simulink model "fused_model"  (R2014b)
settings: Solver=FixedStepAuto  StartTime=0.0  StopTime=100  FixedStep=0.01  RelTol=1e-3
values from neighbouring files (symbols this model uses):
  alpha_AoA = [0 1 2 3 4 5 6 7 8 9 10 11 ... (273 elements, 91x3)]    [alpha_Cd_Cl.mat]    (also in simdata_fused.mat)
  RPM_vs_Throttle = [0 2 4 6 8 10 12 14 16 18 20 22 ... (102 elements, 51x2)]    [RPM_Throttle.mat]    (also in simdata_fused.mat)
  Thrust_vs_PWM = [1100 1110 1120 1130 1140 1150 1160 1170 1180 1190 1200 1210 ... (243 elements, 81x3)]    [Thrust_PWM.mat]    (also in simdata_fused.mat)
  Thrust_vs_RPM = [0 184.4694179 362.7257873 540.6451661 718.059059 894.7989709 1070.696406 1245.58287 1419.289867 1591.648901 1762.491478 1931.649102 ... (102 elements, 51x2)]    [Thrust_RPM.mat]    (also in simdata_fused.mat)
  Torque_vs_RPM = [0 184.4694179 362.7257873 540.6451661 718.059059 894.7989709 1070.696406 1245.58287 1419.289867 1591.648901 1762.491478 1931.649102 ... (102 elements, 51x2)]    [Torque_RPM.mat]    (also in simdata_fused.mat)
libraries: simulink x2
settings Model: Creator=abhij  LastModifiedBy=harsha_home
settings DataIOCC: LimitDataPoints=off  SaveFormat=Dataset
settings OptimizationCC: UseDivisionForNetSlopeComputation=off  SimCompilerOptimization=off
settings DebuggingCC: SolverPrmCheckMsg=none  FrameProcessingCompatibilityMsg=error
settings HardwareCC: ProdBitPerPointer=64  ProdLargestAtomicFloat=Float  ProdIntDivRoundTo=Zero  ProdEndianess=LittleEndian  ProdWordSize=64  ProdHWDeviceType=Intel->x86-64 (Windows64)
settings ModelReferenceCC: PropagateSignalLabelsOutOfModel=on
settings RTWCC: RTWCompilerOptimization=off
settings ConfigComp: CovMetricSettings=dw  CovHtmlReporting=on  CovSaveCumulativeToWorkspaceVar=on  CovSaveSingleToWorkspaceVar=on  CovExternalEMLEnable=off

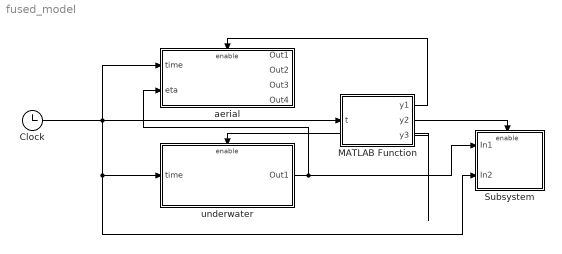
== system fused_model ==
  Clock : Clock
  MATLAB Function : MATLAB Function  TreatAsAtomicUnit=on
  Subsystem : Subsystem
  aerial : Subsystem
  underwater : Subsystem
  wires:
  Clock/1 -> aerial/1(time), Subsystem/2(In2), underwater/1(time), MATLAB Function/1(t)
  MATLAB Function/1(y1) -> aerial/Enable
  underwater/1(Out1) -> Subsystem/1(In1), aerial/2(eta)
  MATLAB Function/3(y3) -> underwater/Enable
  MATLAB Function/2(y2) -> Subsystem/Enable

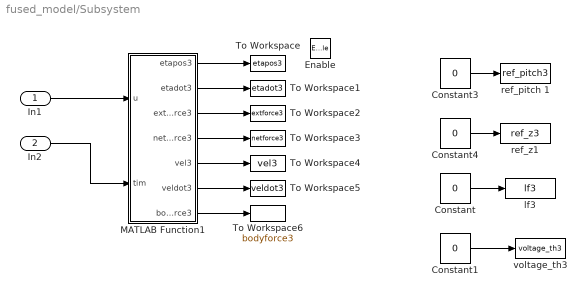
== system fused_model/Subsystem ==
  In1 : Inport
  In2 : Inport  Port=2
  Enable : EnablePort
  Constant{,1,3..4} (4 alike) : Constant  Value=0
  MATLAB Function1 : MATLAB Function  TreatAsAtomicUnit=on
  To Workspace : ToWorkspace  VariableName=etapos3  SaveFormat=Timeseries  SampleTime=-1
  To Workspace1 : ToWorkspace  VariableName=etadot3  SaveFormat=Timeseries  SampleTime=-1
  To Workspace2 : ToWorkspace  VariableName=extforce3  SaveFormat=Timeseries  SampleTime=-1
  To Workspace3 : ToWorkspace  VariableName=netforce3  SaveFormat=Timeseries  SampleTime=-1
  To Workspace4 : ToWorkspace  VariableName=vel3  SaveFormat=Timeseries  SampleTime=-1
  To Workspace5 : ToWorkspace  VariableName=veldot3  SaveFormat=Timeseries  SampleTime=-1
  To Workspace6 : ToWorkspace  VariableName=bodyforce3  SaveFormat=Timeseries  SampleTime=-1
  "lf3 " : ToWorkspace  VariableName=lf3  SaveFormat=Timeseries  SampleTime=-1
  ref_pitch 1 : ToWorkspace  VariableName=ref_pitch3  SaveFormat=Timeseries  SampleTime=-1
  ref_z1 : ToWorkspace  VariableName=ref_z3  SaveFormat=Timeseries  SampleTime=-1
  "voltage_th3 " : ToWorkspace  VariableName=voltage_th3  SaveFormat=Timeseries  SampleTime=-1
  wires:
  In1/1 -> MATLAB Function1/1(u)
  In2/1 -> MATLAB Function1/2(tim)
  MATLAB Function1/1(etapos3) -> To Workspace/1
  MATLAB Function1/2(etadot3) -> To Workspace1/1
  MATLAB Function1/3(extforce3) -> To Workspace2/1
  MATLAB Function1/4(netforce3) -> To Workspace3/1
  MATLAB Function1/5(vel3) -> To Workspace4/1
  MATLAB Function1/6(veldot3) -> To Workspace5/1
  MATLAB Function1/7(bodyforce3) -> To Workspace6/1
  Constant/1 -> "lf3 "/1
  Constant1/1 -> "voltage_th3 "/1
  Constant3/1 -> ref_pitch 1/1
  Constant4/1 -> ref_z1/1

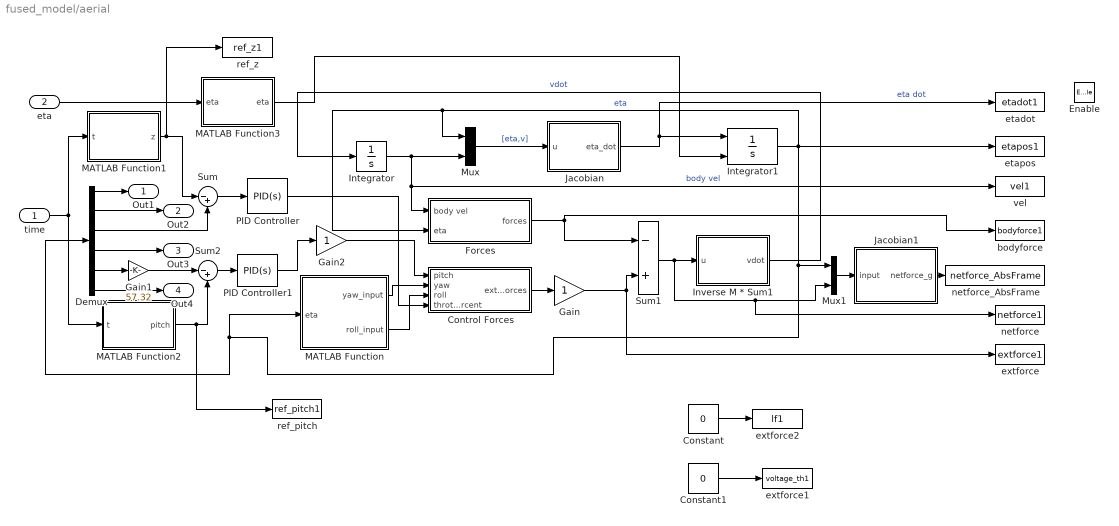
== system fused_model/aerial ==
  time : Inport
  eta : Inport  Port=2
  Enable : EnablePort
  Constant : Constant  Value=0
  Constant1 : Constant  Value=0
  Control Forces : Subsystem
  Demux : Demux  Outputs=6
  Forces : Subsystem
  Gain : Gain
  Gain1 : Gain  Gain=57.32
  Gain2 : Gain
  Integrator : Integrator  InitialCondition=[0;0;0;0;0;0]
  Integrator1 : Integrator  InitialConditionSource=external  InitialCondition=[0;0;0;0;0;0]
  Inverse M * Sum1 : MATLAB Function  TreatAsAtomicUnit=on
  Jacobian : MATLAB Function  TreatAsAtomicUnit=on
  Jacobian1 : MATLAB Function  TreatAsAtomicUnit=on
  MATLAB Function : MATLAB Function  TreatAsAtomicUnit=on
  MATLAB Function1 : MATLAB Function  TreatAsAtomicUnit=on
  MATLAB Function2 : MATLAB Function  TreatAsAtomicUnit=on
  MATLAB Function3 : MATLAB Function  TreatAsAtomicUnit=on
  Mux : Mux  Inputs=2
  Mux1 : Mux  Inputs=2
  PID Controller : simulink/Continuous/PID Controller  Controller=PID  TimeDomain=Continuous-time  SampleTime=-1  IntegratorMethod=Forward Euler  FilterMethod=Forward Euler  Form=Parallel  P=1  I=1  D=0  N=100  InitialConditionSource=internal  InitialConditionForIntegrator=0  InitialConditionForFilter=0  ExternalReset=none  LimitOutput=off  UpperSaturationLimit=inf  LowerSaturationLimit=-inf  LinearizeAsGain=on  AntiWindupMode=none  Kb=1  TrackingMode=off  Kt=1  PParamMin=[]  PParamMax=[]  IParamMin=[]  IParamMax=[]  DParamMin=[]  DParamMax=[]  NParamMin=[]  NParamMax=[]  KbParamMin=[]  KbParamMax=[]  KtParamMin=[]  KtParamMax=[]  POutMin=[]  POutMax=[]  IOutMin=[]  IOutMax=[]  DOutMin=[]  DOutMax=[]  NOutMin=[]  NOutMax=[]  KbOutMin=[]  KbOutMax=[]  KtOutMin=[]  KtOutMax=[]  IntegratorOutMin=[]  IntegratorOutMax=[]  FilterOutMin=[]  FilterOutMax=[]  SumOutMin=[]  SumOutMax=[]  SumI1OutMin=[]  SumI1OutMax=[]  SumI2OutMin=[]  SumI2OutMax=[]  SumI3OutMin=[]  SumI3OutMax=[]  SumDOutMin=[]  SumDOutMax=[]  SaturationOutMin=[]  SaturationOutMax=[]  IntegratorContinuousStateAttributes=''  IntegratorStateMustResolveToSignalObject=off  IntegratorRTWStateStorageClass=Auto  FilterContinuousStateAttributes=''  FilterStateMustResolveToSignalObject=off  FilterRTWStateStorageClass=Auto  DifferentiatorICPrevScaledInput=0  DifferentiatorOutMin=[]  DifferentiatorOutMax=[]  UseFilter=on
  PID Controller1 : simulink/Continuous/PID Controller  Controller=PID  TimeDomain=Continuous-time  SampleTime=-1  IntegratorMethod=Forward Euler  FilterMethod=Forward Euler  Form=Parallel  P=1  I=1  D=0  N=100  InitialConditionSource=internal  InitialConditionForIntegrator=0  InitialConditionForFilter=0  ExternalReset=none  LimitOutput=off  UpperSaturationLimit=inf  LowerSaturationLimit=-inf  LinearizeAsGain=on  AntiWindupMode=none  Kb=1  TrackingMode=off  Kt=1  PParamMin=[]  PParamMax=[]  IParamMin=[]  IParamMax=[]  DParamMin=[]  DParamMax=[]  NParamMin=[]  NParamMax=[]  KbParamMin=[]  KbParamMax=[]  KtParamMin=[]  KtParamMax=[]  POutMin=[]  POutMax=[]  IOutMin=[]  IOutMax=[]  DOutMin=[]  DOutMax=[]  NOutMin=[]  NOutMax=[]  KbOutMin=[]  KbOutMax=[]  KtOutMin=[]  KtOutMax=[]  IntegratorOutMin=[]  IntegratorOutMax=[]  FilterOutMin=[]  FilterOutMax=[]  SumOutMin=[]  SumOutMax=[]  SumI1OutMin=[]  SumI1OutMax=[]  SumI2OutMin=[]  SumI2OutMax=[]  SumI3OutMin=[]  SumI3OutMax=[]  SumDOutMin=[]  SumDOutMax=[]  SaturationOutMin=[]  SaturationOutMax=[]  IntegratorContinuousStateAttributes=''  IntegratorStateMustResolveToSignalObject=off  IntegratorRTWStateStorageClass=Auto  FilterContinuousStateAttributes=''  FilterStateMustResolveToSignalObject=off  FilterRTWStateStorageClass=Auto  DifferentiatorICPrevScaledInput=0  DifferentiatorOutMin=[]  DifferentiatorOutMax=[]  UseFilter=on
  Sum : Sum  Inputs=|-+
  Sum1 : Sum  Inputs=-+
  Sum2 : Sum  Inputs=|-+
  bodyforce : ToWorkspace  VariableName=bodyforce1  SaveFormat=Timeseries  SampleTime=-1
  etadot : ToWorkspace  VariableName=etadot1  SaveFormat=Timeseries  SampleTime=-1
  etapos : ToWorkspace  VariableName=etapos1  SaveFormat=Timeseries  SampleTime=-1
  extforce : ToWorkspace  VariableName=extforce1  SaveFormat=Timeseries  SampleTime=-1
  extforce1 : ToWorkspace  VariableName=voltage_th1  SaveFormat=Timeseries  SampleTime=-1
  extforce2 : ToWorkspace  VariableName=lf1  SaveFormat=Timeseries  SampleTime=-1
  netforce : ToWorkspace  VariableName=netforce1  SaveFormat=Timeseries  SampleTime=-1
  netforce_AbsFrame : ToWorkspace  VariableName=netforce_AbsFrame  SaveFormat=Timeseries  SampleTime=-1
  "ref_pitch " : ToWorkspace  VariableName=ref_pitch1  SaveFormat=Timeseries  SampleTime=-1
  ref_z : ToWorkspace  VariableName=ref_z1  SaveFormat=Timeseries  SampleTime=-1
  vel : ToWorkspace  VariableName=vel1  SaveFormat=Timeseries  SampleTime=-1
  Out1 : Outport
  Out2 : Outport  Port=2
  Out3 : Outport  Port=3
  Out4 : Outport  Port=4
  wires:
  MATLAB Function/1(yaw_input) -> Control Forces/2(yaw)
  time/1 -> MATLAB Function2/1(t), MATLAB Function1/1(t)
  Jacobian/1(eta_dot) -> etadot/1, Integrator1/1  "eta dot"
  Gain2/1 -> Control Forces/1(pitch)
  MATLAB Function/2(roll_input) -> Control Forces/3(roll)
  PID Controller1/1 -> Gain2/1
  Demux/3 -> Sum/2
  Sum1/1 -> netforce/1, Mux1/2, Inverse M * Sum1/1(u)
  MATLAB Function2/1(pitch) -> "ref_pitch "/1, Sum2/2
  PID Controller/1 -> Control Forces/4(throttle percent)
  Jacobian1/1(netforce_g) -> netforce_AbsFrame/1
  Sum2/1 -> PID Controller1/1
  Mux/1 -> Jacobian/1(u)  "[eta,v]"
  Gain/1 -> extforce/1, Sum1/2
  MATLAB Function1/1(z) -> ref_z/1, Sum/1
  Control Forces/1(external forces) -> Gain/1
  Sum/1 -> PID Controller/1
  Integrator/1 -> vel/1, Forces/1(body vel), Mux/2  "body vel"
  Integrator1/1 -> Forces/2(eta), Mux/1, Demux/1, MATLAB Function/1(eta), Mux1/1, etapos/1  "eta"
  Forces/1(forces) -> Sum1/1, bodyforce/1
  Mux1/1 -> Jacobian1/1(input)
  Demux/5 -> Gain1/1
  Gain1/1 -> Sum2/1
  eta/1 -> MATLAB Function3/1("eta ")
  Inverse M * Sum1/1(vdot) -> Integrator/1  "vdot"
  Demux/1 -> Out1/1
  Demux/2 -> Out2/1
  Demux/4 -> Out3/1
  Demux/6 -> Out4/1
  MATLAB Function3/1(eta) -> Integrator1/2
  Constant/1 -> extforce2/1
  Constant1/1 -> extforce1/1

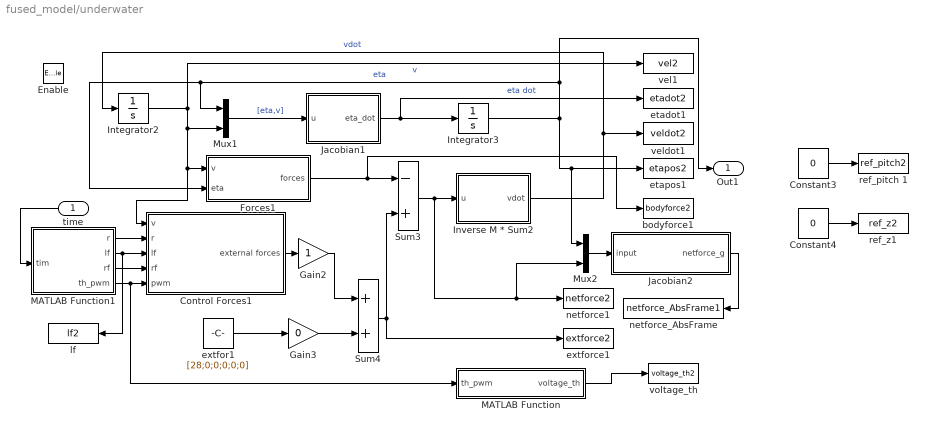
== system fused_model/underwater ==
  time : Inport
  Enable : EnablePort
  Constant3 : Constant  Value=0
  Constant4 : Constant  Value=0
  Control Forces1 : Subsystem
  Forces1 : Subsystem
  Gain2 : Gain
  Gain3 : Gain  Gain=0
  Integrator2 : Integrator  InitialCondition=[0;0;0;0;0;0]
  Integrator3 : Integrator  InitialCondition=[0;0;5;0;0;0]
  Inverse M * Sum2 : MATLAB Function  TreatAsAtomicUnit=on
  Jacobian1 : MATLAB Function  TreatAsAtomicUnit=on
  Jacobian2 : MATLAB Function  TreatAsAtomicUnit=on
  MATLAB Function : MATLAB Function  TreatAsAtomicUnit=on
  MATLAB Function1 : MATLAB Function  TreatAsAtomicUnit=on
  Mux1 : Mux  Inputs=2
  Mux2 : Mux  Inputs=2
  Sum3 : Sum  Inputs=-+
  Sum4 : Sum
  bodyforce1 : ToWorkspace  VariableName=bodyforce2  SaveFormat=Timeseries  SampleTime=-1
  etadot1 : ToWorkspace  VariableName=etadot2  SaveFormat=Timeseries  SampleTime=-1
  etapos1 : ToWorkspace  VariableName=etapos2  SaveFormat=Timeseries  SampleTime=-1
  extfor1 : Constant  Value=[28;0;0;0;0;0]
  extforce1 : ToWorkspace  VariableName=extforce2  SaveFormat=Timeseries  SampleTime=-1
  lf : ToWorkspace  VariableName=lf2  SaveFormat=Timeseries  SampleTime=-1
  netforce1 : ToWorkspace  VariableName=netforce2  SaveFormat=Timeseries  SampleTime=-1
  netforce_AbsFrame : ToWorkspace  VariableName=netforce_AbsFrame1  SaveFormat=Timeseries  SampleTime=-1
  ref_pitch 1 : ToWorkspace  VariableName=ref_pitch2  SaveFormat=Timeseries  SampleTime=-1
  ref_z1 : ToWorkspace  VariableName=ref_z2  SaveFormat=Timeseries  SampleTime=-1
  vel1 : ToWorkspace  VariableName=vel2  SaveFormat=Timeseries  SampleTime=-1
  veldot1 : ToWorkspace  VariableName=veldot2  SaveFormat=Timeseries  SampleTime=-1
  "voltage_th " : ToWorkspace  VariableName=voltage_th2  SaveFormat=Timeseries  SampleTime=-1
  Out1 : Outport
  wires:
  Integrator2/1 -> vel1/1, Forces1/1(v), Control Forces1/1(v), Mux1/2  "v"
  Mux1/1 -> Jacobian1/1(u)  "[eta,v]"
  Jacobian1/1(eta_dot) -> etadot1/1, Integrator3/1  "eta dot"
  Integrator3/1 -> Mux2/1, etapos1/1, Out1/1, Forces1/2(eta), Mux1/1  "eta"
  Sum3/1 -> netforce1/1, Mux2/2, Inverse M * Sum2/1(u)
  Forces1/1(forces) -> Sum3/1, bodyforce1/1
  Control Forces1/1(external forces) -> Gain2/1
  Gain2/1 -> Sum4/1
  Gain3/1 -> Sum4/2
  extfor1/1 -> Gain3/1
  Sum4/1 -> Sum3/2, extforce1/1
  Mux2/1 -> Jacobian2/1(input)
  Jacobian2/1(netforce_g) -> netforce_AbsFrame/1
  Inverse M * Sum2/1(vdot) -> Integrator2/1, veldot1/1  "vdot"
  MATLAB Function1/1(r) -> Control Forces1/2(r)
  MATLAB Function1/2(lf) -> Control Forces1/3(lf), lf/1
  MATLAB Function1/3(rf) -> Control Forces1/4(rf)
  time/1 -> MATLAB Function1/1(tim)
  MATLAB Function1/4(th_pwm) -> MATLAB Function/1(th_pwm), Control Forces1/5("pwm ")
  MATLAB Function/1(voltage_th) -> "voltage_th "/1
  Constant3/1 -> ref_pitch 1/1
  Constant4/1 -> ref_z1/1

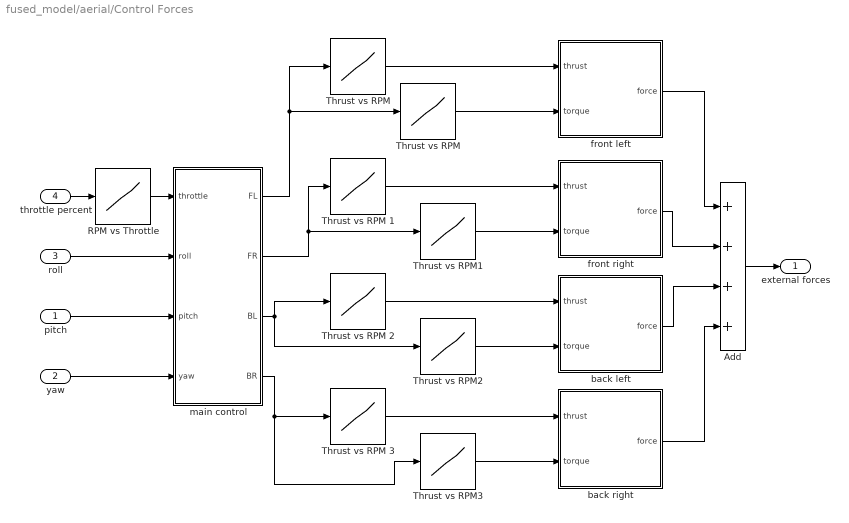
== system fused_model/aerial/Control Forces ==
  pitch : Inport
  yaw : Inport  Port=2
  roll : Inport  Port=3
  throttle percent : Inport  Port=4
  Add : Sum  Inputs=4
  "RPM vs Throttle " : Lookup_n-D  NumberOfTableDimensions=1  BreakpointsForDimension1=RPM_vs_Throttle(:,1)  Table=RPM_vs_Throttle(:,2)  InternalRulePriority=Speed  RndMeth=Simplest  InputSameDT=on
  Thrust vs RPM{,1..3} (4 alike) : Lookup_n-D  NumberOfTableDimensions=1  BreakpointsForDimension1=Torque_vs_RPM(:,1)  Table=Torque_vs_RPM(:,2)  InternalRulePriority=Speed  RndMeth=Simplest  InputSameDT=on
  Thrust vs RPM {,1..3} (4 alike) : Lookup_n-D  NumberOfTableDimensions=1  BreakpointsForDimension1=Thrust_vs_RPM(:,1)  Table=Thrust_vs_RPM(:,2)  InternalRulePriority=Speed  RndMeth=Simplest  InputSameDT=on
  back left : MATLAB Function  TreatAsAtomicUnit=on
  back right : MATLAB Function  TreatAsAtomicUnit=on
  front left : MATLAB Function  TreatAsAtomicUnit=on
  front right : MATLAB Function  TreatAsAtomicUnit=on
  main control : MATLAB Function  TreatAsAtomicUnit=on
  external forces : Outport
  wires:
  front left/1(force) -> Add/1
  front right/1(force) -> Add/2
  back left/1(force) -> Add/3
  back right/1(force) -> Add/4
  main control/1(FL) -> Thrust vs RPM/1, "Thrust vs RPM "/1
  main control/2(FR) -> Thrust vs RPM 1/1, Thrust vs RPM1/1
  main control/3(BL) -> Thrust vs RPM2/1, Thrust vs RPM 2/1
  main control/4(BR) -> Thrust vs RPM3/1, Thrust vs RPM 3/1
  throttle percent/1 -> "RPM vs Throttle "/1
  roll/1 -> main control/2(roll)
  pitch/1 -> main control/3(pitch)
  yaw/1 -> main control/4(yaw)
  "RPM vs Throttle "/1 -> main control/1(throttle)
  Thrust vs RPM/1 -> front left/2(torque)
  Thrust vs RPM1/1 -> front right/2(torque)
  Thrust vs RPM2/1 -> back left/2(torque)
  Thrust vs RPM3/1 -> back right/2(torque)
  "Thrust vs RPM "/1 -> front left/1(thrust)
  Thrust vs RPM 1/1 -> front right/1(thrust)
  Thrust vs RPM 2/1 -> back left/1(thrust)
  Thrust vs RPM 3/1 -> back right/1(thrust)
  Add/1 -> external forces/1

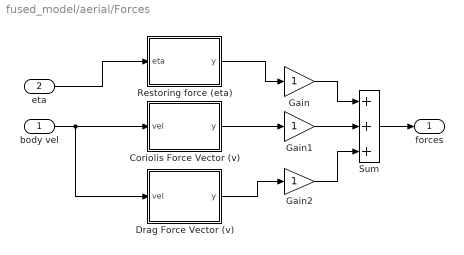
== system fused_model/aerial/Forces ==
  body vel : Inport
  eta : Inport  Port=2
  Coriolis Force Vector (v) : MATLAB Function  TreatAsAtomicUnit=on
  Drag Force Vector (v) : MATLAB Function  TreatAsAtomicUnit=on
  Gain : Gain
  Gain1 : Gain
  Gain2 : Gain
  Restoring force (eta) : MATLAB Function  TreatAsAtomicUnit=on
  Sum : Sum  Inputs=+++
  forces : Outport
  wires:
  Restoring force (eta)/1(y) -> Gain/1
  Coriolis Force Vector (v)/1(y) -> Gain1/1
  Drag Force Vector (v)/1(y) -> Gain2/1
  Sum/1 -> forces/1
  body vel/1 -> Drag Force Vector (v)/1(vel), Coriolis Force Vector (v)/1(vel)
  eta/1 -> Restoring force (eta)/1(eta)
  Gain1/1 -> Sum/2
  Gain/1 -> Sum/1
  Gain2/1 -> Sum/3

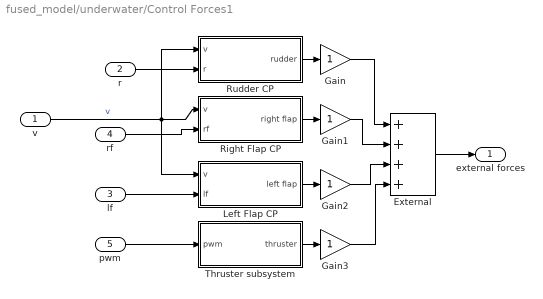
== system fused_model/underwater/Control Forces1 ==
  v : Inport
  r : Inport  Port=2
  lf : Inport  Port=3
  rf : Inport  Port=4
  "pwm " : Inport  Port=5
  "External " : Sum  Inputs=++++
  Gain{,1..3} (4 alike) : Gain
  Left Flap CP : Subsystem
  Right Flap CP : Subsystem
  Rudder CP : Subsystem
  Thruster subsystem : Subsystem
  external forces : Outport
  wires:
  v/1 -> Rudder CP/1(v), Left Flap CP/1(v), Right Flap CP/1(v)  "v"
  Rudder CP/1("rudder ") -> Gain/1
  "External "/1 -> external forces/1
  Gain/1 -> "External "/1
  Right Flap CP/1(right flap) -> Gain1/1
  Gain1/1 -> "External "/2
  Left Flap CP/1(left flap) -> Gain2/1
  Gain2/1 -> "External "/3
  Thruster subsystem/1(thruster) -> Gain3/1
  Gain3/1 -> "External "/4
  r/1 -> Rudder CP/2(r)
  rf/1 -> Right Flap CP/2(rf)
  lf/1 -> Left Flap CP/2(lf)
  "pwm "/1 -> Thruster subsystem/1(pwm)

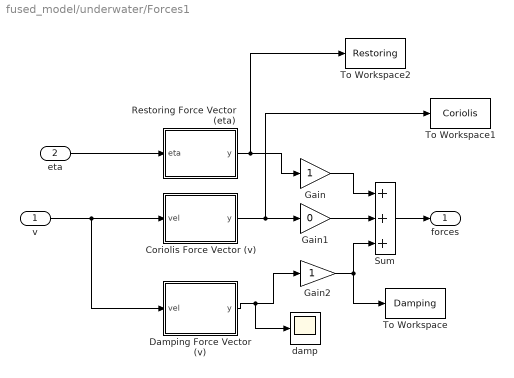
== system fused_model/underwater/Forces1 ==
  v : Inport
  eta : Inport  Port=2
  Coriolis Force Vector (v) : MATLAB Function  TreatAsAtomicUnit=on
  Damping Force Vector (v) : MATLAB Function  TreatAsAtomicUnit=on
  Gain : Gain
  Gain1 : Gain  Gain=0
  Gain2 : Gain
  Restoring Force Vector (eta) : MATLAB Function  TreatAsAtomicUnit=on
  Sum : Sum  Inputs=+++
  To Workspace : ToWorkspace  VariableName=Damping  SaveFormat=Timeseries  SampleTime=-1
  To Workspace1 : ToWorkspace  VariableName=Coriolis  SaveFormat=Timeseries  SampleTime=-1
  To Workspace2 : ToWorkspace  VariableName=Restoring  SaveFormat=Timeseries  SampleTime=-1
  damp : Scope
  forces : Outport
  wires:
  Restoring Force Vector (eta)/1(y) -> To Workspace2/1, Gain/1
  Coriolis Force Vector (v)/1(y) -> To Workspace1/1, Gain1/1
  Damping Force Vector (v)/1(y) -> damp/1, Gain2/1
  Sum/1 -> forces/1
  v/1 -> Damping Force Vector (v)/1(vel), Coriolis Force Vector (v)/1(vel)
  eta/1 -> Restoring Force Vector (eta)/1(eta)
  Gain1/1 -> Sum/2
  Gain/1 -> Sum/1
  Gain2/1 -> Sum/3, To Workspace/1

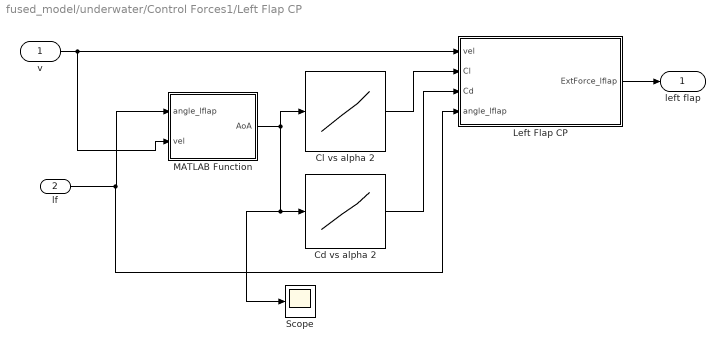
== system fused_model/underwater/Control Forces1/Left Flap CP ==
  v : Inport
  lf : Inport  Port=2
  Cd vs alpha 2 : Lookup_n-D  NumberOfTableDimensions=1  BreakpointsForDimension1=alpha_AoA(:,1)  Table=alpha_AoA(:,2)  InternalRulePriority=Speed  RndMeth=Simplest  InputSameDT=on
  Cl vs alpha 2 : Lookup_n-D  NumberOfTableDimensions=1  BreakpointsForDimension1=alpha_AoA(:,1)  Table=alpha_AoA(:,3)  InternalRulePriority=Speed  RndMeth=Simplest  InputSameDT=on
  Left Flap CP : MATLAB Function  TreatAsAtomicUnit=on
  MATLAB Function : MATLAB Function  TreatAsAtomicUnit=on
  Scope : Scope
  left flap : Outport
  wires:
  v/1 -> Left Flap CP/1(vel), MATLAB Function/2(vel)
  Left Flap CP/1(ExtForce_lflap) -> left flap/1
  Cl vs alpha 2/1 -> Left Flap CP/2(Cl)
  Cd vs alpha 2/1 -> Left Flap CP/3(Cd)
  MATLAB Function/1(AoA) -> Cl vs alpha 2/1, Scope/1, Cd vs alpha 2/1
  lf/1 -> Left Flap CP/4(angle_lflap), MATLAB Function/1(angle_lflap)

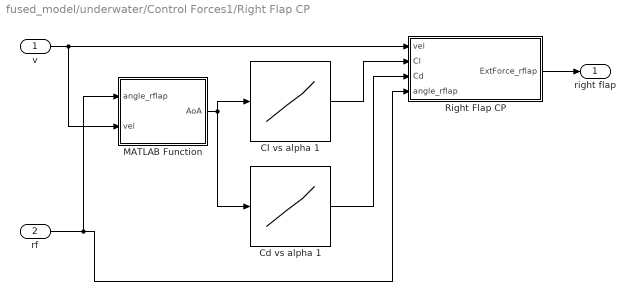
== system fused_model/underwater/Control Forces1/Right Flap CP ==
  v : Inport
  rf : Inport  Port=2
  Cd vs alpha 1 : Lookup_n-D  NumberOfTableDimensions=1  BreakpointsForDimension1=alpha_AoA(:,1)  Table=alpha_AoA(:,2)  InternalRulePriority=Speed  RndMeth=Simplest  InputSameDT=on
  Cl vs alpha 1 : Lookup_n-D  NumberOfTableDimensions=1  BreakpointsForDimension1=alpha_AoA(:,1)  Table=alpha_AoA(:,3)  InternalRulePriority=Speed  RndMeth=Simplest  InputSameDT=on
  MATLAB Function : MATLAB Function  TreatAsAtomicUnit=on
  Right Flap CP : MATLAB Function  TreatAsAtomicUnit=on
  right flap : Outport
  wires:
  v/1 -> Right Flap CP/1(vel), MATLAB Function/2(vel)
  Right Flap CP/1(ExtForce_rflap) -> right flap/1
  Cl vs alpha 1/1 -> Right Flap CP/2(Cl)
  Cd vs alpha 1/1 -> Right Flap CP/3(Cd)
  rf/1 -> Right Flap CP/4(angle_rflap), MATLAB Function/1(angle_rflap)
  MATLAB Function/1(AoA) -> Cd vs alpha 1/1, Cl vs alpha 1/1

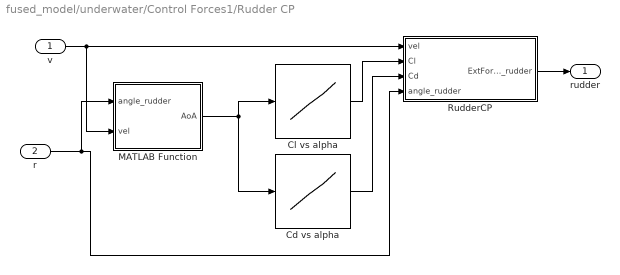
== system fused_model/underwater/Control Forces1/Rudder CP ==
  v : Inport
  r : Inport  Port=2
  "Cd vs alpha " : Lookup_n-D  NumberOfTableDimensions=1  BreakpointsForDimension1=alpha_AoA(:,1)  Table=alpha_AoA(:,2)  InternalRulePriority=Speed  RndMeth=Simplest  InputSameDT=on
  "Cl vs alpha " : Lookup_n-D  NumberOfTableDimensions=1  BreakpointsForDimension1=alpha_AoA(:,1)  Table=alpha_AoA(:,3)  InternalRulePriority=Speed  RndMeth=Simplest  InputSameDT=on
  MATLAB Function : MATLAB Function  TreatAsAtomicUnit=on
  "RudderCP " : MATLAB Function  TreatAsAtomicUnit=on
  "rudder " : Outport
  wires:
  v/1 -> "RudderCP "/1(vel), MATLAB Function/2(vel)
  "RudderCP "/1(ExtForce_rudder) -> "rudder "/1
  "Cl vs alpha "/1 -> "RudderCP "/2(Cl)
  "Cd vs alpha "/1 -> "RudderCP "/3(Cd)
  MATLAB Function/1(AoA) -> "Cl vs alpha "/1, "Cd vs alpha "/1
  r/1 -> MATLAB Function/1(angle_rudder), "RudderCP "/4(angle_rudder)

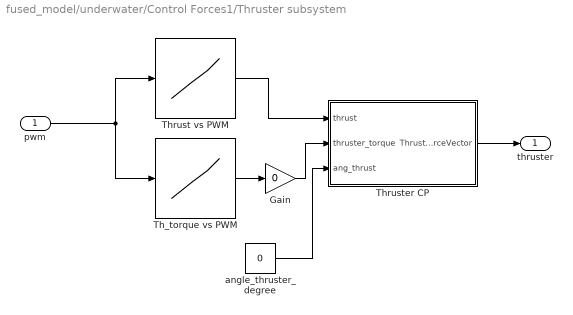
== system fused_model/underwater/Control Forces1/Thruster subsystem ==
  pwm : Inport
  Gain : Gain  Gain=0
  Th_torque vs PWM : Lookup_n-D  NumberOfTableDimensions=1  BreakpointsForDimension1=Thrust_vs_PWM(:,1)  BreakpointsForDimension2=Thrust_vs_PWM(:,3)  Table=Thrust_vs_PWM(:,3)  InternalRulePriority=Speed  RndMeth=Simplest  InputSameDT=on
  Thrust vs PWM : Lookup_n-D  NumberOfTableDimensions=1  BreakpointsForDimension1=Thrust_vs_PWM(:,1)  BreakpointsForDimension2=Thrust_vs_PWM(:,3)  Table=Thrust_vs_PWM(:,2)  InternalRulePriority=Speed  RndMeth=Simplest  InputSameDT=on
  Thruster CP : MATLAB Function  TreatAsAtomicUnit=on
  angle_thruster_degree : Constant  Value=0
  thruster : Outport
  wires:
  Thruster CP/1(ThrusterForceVector) -> thruster/1
  angle_thruster_degree/1 -> Thruster CP/3(ang_thrust)
  Thrust vs PWM/1 -> Thruster CP/1(thrust)
  Th_torque vs PWM/1 -> Gain/1
  Gain/1 -> Thruster CP/2(thruster_torque)
  pwm/1 -> Th_torque vs PWM/1, Thrust vs PWM/1

== matlab function fused_model/aerial/MATLAB Function3 ==
  data: eta input; eta output
function eta = fcn(eta)

eta(2)=0;
eta(3)=0;
eta(4)=0;
eta(5)=0;
eta(6)=0;
end

== matlab function fused_model/Subsystem/MATLAB Function1 ==
  data: u input; etapos3 output; etadot3 output; extforce3 output; netforce3 output; vel3 output; veldot3 output; bodyforce3 output; tim input
function [etapos3,etadot3,extforce3,netforce3,vel3,veldot3,bodyforce3]= fcn(u,tim)
etapos3=u;
etadot3=[0;0;0;0;0;0];
extforce3=[0;0;0;0;0;0];
netforce3=[0;0;0;0;0;0];
vel3=[0;0;0;0;0;0];
veldot3=[0;0;0;0;0;0];
bodyforce3=[0;0;0;0;0;0];
end

== matlab function fused_model/underwater/MATLAB Function ==
  data: th_pwm input; voltage_th output
function voltage_th = fcn(th_pwm)

voltage_th = 16*(th_pwm - 1500)/400;

end

== matlab function fused_model/aerial/Control Forces/back left ==
  data: thrust input; force output; torque input
function force = fcn(thrust,torque)
l=0.500;
b=0.600;
force=[ 0;
        0;
        -thrust;
        -thrust*b/2;
        -thrust*l/2;
        -torque];
end

== matlab function fused_model/aerial/Control Forces/back right ==
  data: thrust input; force output; torque input
function force = fcn(thrust,torque)
l=0.500;
b=0.600;
force=[ 0;
        0;
        -thrust;
        thrust*b/2;
        -thrust*l/2;
        torque];
end

== matlab function fused_model/aerial/Control Forces/front left ==
  data: thrust input; force output; torque input
function force = fcn(thrust,torque)
l=0.500;
b=0.600;
force=[ 0;
        0;
        -thrust;
        -thrust*b/2;
        thrust*l/2;
        torque];
end

== matlab function fused_model/aerial/Control Forces/front right ==
  data: thrust input; force output; torque input
function force = fcn(thrust,torque)
l=0.500;
b=0.600;

force=[ 0;
        0;
        -thrust;
        thrust*b/2;
        thrust*l/2;
        -torque];
end

== matlab function fused_model/aerial/Control Forces/main control ==
  data: throttle input; FL output; roll input; pitch input; yaw input; FR output; BL output; BR output
function [FL,FR,BL,BR]= fcn(throttle,roll,pitch,yaw)
pitchmax = 37.4; %degrees
rollmax  = 40.7;
yawmax = 0.6825;
RPM_max=6270;

%pitch= pitch/pitchmax;
roll= roll/rollmax;
yaw= yaw*yawmax;
throttle=throttle; %in RPM
a=1;%throttle coeff
b=1;%pitch coeff
c=.03;%roll coeff
d=.02;%yaw coeff

FL = throttle*a + RPM_max*(pitch*b+roll*c+yaw*d);
FR = throttle*a + RPM_max*(pitch*b-roll*c-yaw*d);
BL = throttle*a + RPM_max*(-pitch*b+roll*c-yaw*d);
BR = throttle*a + RPM_max*(-pitch*b-roll*c+yaw*d);

if FL>RPM_max
    FL=RPM_max;
end
if FR>RPM_max
    FR=RPM_max;
end    
if BL>RPM_max
    BL=RPM_max;
end    
if BR>RPM_max
    BR=RPM_max;
end    

end

== matlab function fused_model/aerial/Forces/Coriolis Force Vector (v) ==
  data: vel input; y output
function y = fcn(vel)
u = vel(1);
v = vel(2);
w = vel(3);
p = vel(4);
q = vel(5);
r = vel(6);
m = 7;
Iz = 0.157;
Ix = 0.037;
Iy = 0.164;
xg = 0;
zg = 0.090;

C_rb=[0                0              0          m*zg*r    m*(w-xg*q)    -m*(v+xg*r);
      0                0              0         -m*w     m*(zg*r +xg*p)     m*u;
      0                0              0          m*v      -m*(zg*q+u)      m*xg*p;
    -m*zg*r           m*w        m*(zg*p-v)      0           Iz*r         -Iy*q;
   m*(xg*q-w)  -m*(zg*r +xg*p)  m*(zg*q+u)     -Iz*r          0            Ix*p;
   m*(v+xg*r)       -m*u         -m*xg*p       Iy*q          -Ix*p          0      ];
  
% XU = -.7;
% YV = -6.952;
% ZW = -6.952;
% KP = 0;
% MQ = -0.22;
% NR = -0.22;
% 
% C_a =  [0       0       0       0       -ZW*w   YV*v;
%         0       0       0       ZW*w    0       -XU*u;
%         0       0       0       -YV*v   XU*u    0;
%         0       -ZW*w   YV*v    0       -NR*r   MQ*q;
%         ZW*w    0       -XU*u   NR*r    0       -KP*p;
%         -YV*v   XU*u    0       -MQ*q   KP*p       0];
   
C = C_rb;
y = C*vel;
end

== matlab function fused_model/aerial/Forces/Drag Force Vector (v) ==
  data: vel input; y output
function y = fcn(vel)
u = vel(1);
v = vel(2);
w = vel(3);
p = vel(4);
q = vel(5);
r = vel(6);



y=2*[1/30*u*abs(u); 
   4/30*v*abs(v);
   4/30*w*abs(w);
   2/100*p*abs(p);
   30/100*q*abs(q);
   4/100*r*abs(r);];
end

== matlab function fused_model/aerial/Forces/Restoring force (eta) ==
  data: eta input; y output
function y = fcn(eta)

theta = eta(5);
phi = eta(4);

W=7*9.81;
Xg=0;
Zg=0.090;

G=   [ W*sin(theta);
       -W*cos(theta)*sin(phi);
       -W*cos(theta)*cos(phi);
       Zg*W*cos(theta)*sin(phi);
       Zg*W*sin(theta);
       0];
y =  G;

% for simulation Zb=Zg assumed
%       x           y   z
%cog	-301.22		0	89.16	(weight  ~6.8 kgs)
%cob	-308.44		0	96.30   (buoyancy 7.8 kgs)
end

== matlab function fused_model/aerial/Inverse M * Sum1 ==
  data: u input; vdot output
function vdot = fcn(u)
sum1 = u;
xg = 0;
zg = 0.090;
m = 7;
I=m*zg^2;
M_rb=[m     0      0     0       m*zg      0;
      0     m      0     -m*zg    0        m*xg;
      0     0      m     0       -m*xg        0;
      0    m*zg    0    0.037+I        0        0;
      m*zg  0     -m*xg     0    0.164+I    0;
      0    m*xg      0     0       0      0.157];

% M_a= -1*[-0.m   0       0       0       0       0;
%         0      -6.952  0       0       0       0;    
%         0      0       -6.952  0       0       0;
%         0      0       0       0       0       0;
%         0      0       0       0       -0.22   0;
%         0      0       0       0       0       -0.22];

% equivalent cylinder dimension r=.06 l=.615  
M=M_rb; 
vdot = inv(M)*sum1;
end

== matlab function fused_model/aerial/Jacobian ==
  data: u input; eta_dot output
function eta_dot = fcn(u)

v = u(7:12); %body_frame_velocities

phi=u(4); %roll
theta=u(5); %pitch
si=u(6);   %yaw
c_p=cos(phi);
c_t=cos(theta);
c_s=cos(si);
s_p=sin(phi);
s_t=sin(theta);
s_s=sin(si);
t_t=tan(theta);


J1=[c_s*c_t    -s_s*c_p+s_p*s_t*c_s     s_s*s_p+s_t*c_s*c_p;
    s_s*c_t     c_s*c_p+s_p*s_t*s_s    -c_s*s_p+s_t*s_s*c_p;
     -s_t            s_p*c_t                 c_p*c_t       ];
       
J2=[1      s_p*t_t     c_p*t_t;
    0        c_p        -s_p;
    0      s_p/c_t     c_p/c_t ];


J=[J1 zeros(3,3); zeros(3,3) J2];
eta_dot = J * v; % y == earth_velocities

end

== matlab function fused_model/aerial/Jacobian1 ==
  data: input input; netforce_g output
function netforce_g = fcn(input)

netforce_b = input(7:12); %body_frame_velocities

phi=input(4); %roll
theta=input(5); %pitch
si=input(6);   %yaw
c_p=cos(phi);
c_t=cos(theta);
c_s=cos(si);
s_p=sin(phi);
s_t=sin(theta);
s_s=sin(si);
t_t=tan(theta);


J1=[c_s*c_t    -s_s*c_p+s_p*s_t*c_s     s_s*s_p+s_t*c_s*c_p;
    s_s*c_t     c_s*c_p+s_p*s_t*s_s    -c_s*s_p+s_t*s_s*c_p;
     -s_t            s_p*c_t                 c_p*c_t       ];
       
J2=[1      s_p*t_t     c_p*t_t;
    0        c_p        -s_p;
    0      s_p/c_t     c_p/c_t ];


J=[J1 zeros(3,3); zeros(3,3) J2];
netforce_g = J * netforce_b; % y == earth_velocities

end

== matlab function fused_model/aerial/MATLAB Function ==
  data: yaw_input output; roll_input output; eta input
function [yaw_input,roll_input] = fcn(eta)

kp=0;
ki=0;
kd=0;

pitch_reference=0;
z_reference=0;

pitch_input=0;
yaw_input=0;
roll_input=0;
throttle_input=64.835;
end

== matlab function fused_model/aerial/MATLAB Function1 ==
  data: t input; z output
function z = fcn(t)

ini_z=0;
z=ini_z-2*(t-50);
if z<-20
    z=-20;
end

end

== matlab function fused_model/aerial/MATLAB Function2 ==
  data: t input; pitch output
function pitch = fcn(t)

% ini_z=0;
% z=ini_z+10*t;
% if z>0
%     z=0;
% end
pitch=-5;
end

== matlab function fused_model/MATLAB Function ==
  data: y1 output; y2 output; t input; y3 output
function [y1,y2,y3] = fcn(t)


if t>50
    y1=1;
    y2=0;
    y3=0;
elseif t<=50 && t>45.36
    y1=0;
    y2=1;
    y3=0;
else
    y1=0;
    y2=0;
    y3=1;
end
end

== matlab function fused_model/underwater/Control Forces1/Left Flap CP/Left Flap CP ==
  data: vel input; ExtForce_lflap output; Cl input; Cd input; angle_lflap input
function ExtForce_lflap = fcn(vel,Cl,Cd,angle_lflap)

l=0;
d=0;
u = vel(1);
w = vel(3);

angle1 = angle_lflap*pi/180;
angle_rad = atan2(w,u);
u0 = u*cos(angle1)-w*sin(angle1);
w0 = u*sin(angle1)+w*cos(angle1);

rho = 1000;

A_lflap = 0.02075;
a = 0.100; b= 0.150; rx = 0.090; rz = 0.030; ry = 0.088;

V = sqrt(u^2+w^2);
%%

if u0>=0 && w0>=0
   d=1;
   l=1;
elseif u0>=0 && w0<0
   d=1;
   l=-1;
elseif u0<0 && w0<0
   d=1;
   l=-1;
elseif u0>=0 && w0<0
   d=1;
   l=1;
end
%%
L = l*(1/2)*Cl*rho*A_lflap*V*V;
D = d*(1/2)*Cd*rho*A_lflap*V*V;
Fx = -D*cos(angle_rad)+L*sin(angle_rad);
Fy =  0;
Fz =  -(D*sin(angle_rad)+L*cos(angle_rad));
Mx = -(Fz*(ry+(a/2)));
My =  Fx*(rz+(b/2)*sin(angle_rad))+Fz*(rx+(b/2)*cos(angle_rad));
Mz = -(Fx*(ry+(a/2)));

ExtForce_lflap = [Fx;Fy;Fz;Mx;My;Mz];

end

== matlab function fused_model/underwater/Control Forces1/Left Flap CP/MATLAB Function ==
  data: angle_lflap input; AoA output; vel input
function AoA= fcn(angle_lflap,vel)
%#codegen
u = vel(1);
w = vel(3);
angle_rad = angle_lflap*pi/180;
u0 = u*cos(angle_rad)-w*sin(angle_rad);
w0 = u*sin(angle_rad)+w*cos(angle_rad);

alpha = abs(atan2(w0,u0));
AoA=alpha;

end

== matlab function fused_model/underwater/Control Forces1/Right Flap CP/MATLAB Function ==
  data: angle_rflap input; vel input; AoA output
function AoA = fcn(angle_rflap,vel)
%#codegen
u = vel(1);
w = vel(3);
angle_rad = angle_rflap*pi/180;
u0 = u*cos(angle_rad)-w*sin(angle_rad);
w0 = u*sin(angle_rad)+w*cos(angle_rad);

alpha = abs(atan2(w0,u0));
AoA=alpha;

end

== matlab function fused_model/underwater/Control Forces1/Right Flap CP/Right Flap CP ==
  data: vel input; ExtForce_rflap output; Cl input; Cd input; angle_rflap input
function ExtForce_rflap = fcn(vel,Cl,Cd,angle_rflap)

l=0;
d=0;

u = vel(1);
w = vel(3);
rho = 1000;

angle1 = angle_rflap*pi/180;
angle_rad = atan2(w,u);
u0 = u*cos(angle1)-w*sin(angle1);
w0 = u*sin(angle1)+w*cos(angle1);

V = sqrt(u^2+w^2);

A_rflap = 0.02075;
a = 0.100; b= 0.150; rx = 0.090; rz = 0.030; ry = 0.088;
%%

if u0>=0 && w0>=0
   d=1;
   l=1;
elseif u0>=0 && w0<0
   d=1;
   l=-1;
elseif u0<0 && w0<0
   d=1;
   l=-1;
elseif u0>=0 && w0<0
   d=1;
   l=1;
end
%%
L = l*(1/2)*Cl*rho*A_rflap*V*V;
D = d*(1/2)*Cd*rho*A_rflap*V*V;
Fx = -D*cos(angle_rad)+L*sin(angle_rad);
Fy =  0;
Fz =  -(D*sin(angle_rad)+L*cos(angle_rad));
Mx =  Fz*(ry+(a/2));
My =  Fx*(rz+(b/2)*sin(angle_rad))+Fz*(rx+(b/2)*cos(angle_rad));
Mz =  Fx*(ry+(a/2));

ExtForce_rflap = [Fx;Fy;Fz;Mx;My;Mz];

end

== matlab function fused_model/underwater/Control Forces1/Rudder CP/MATLAB Function ==
  data: angle_rudder input; AoA output; vel input
function AoA = fcn(angle_rudder,vel)
%#codegen
u = vel(1);
v = vel(2);

angle_rad = angle_rudder*pi/180;
u0 = u*cos(angle_rad)-v*sin(angle_rad);
v0 = u*sin(angle_rad)+v*cos(angle_rad);

alpha = abs(atan2(v0,u0));
AoA=alpha;
end

== matlab function fused_model/underwater/Control Forces1/Rudder CP/RudderCP  ==
  data: vel input; ExtForce_rudder output; Cl input; Cd input; angle_rudder input
function ExtForce_rudder = fcn(vel,Cl,Cd,angle_rudder)
l=0;
d=0;
u = vel(1);
v = vel(2);
rho = 1000;

angle1 = angle_rudder*pi/180;
angle_rad = atan2(v,u);
u0 = u*cos(angle1)-v*sin(angle1);
v0 = u*sin(angle1)+v*cos(angle1);

V = sqrt(u^2+v^2);
%%

if u0>=0 && v0>=0
   d=1;
   l=1;
elseif u0>=0 && v0<0
   d=1;
   l=-1;
elseif u0<0 && v0<0
   d=1;
   l=-1;
elseif u0>=0 && v0<0
   d=1;
   l=1;
end
%%
A_rudder = 0.01;
a = 0.1; b= 0.1; rx = 0.135; rz =0.06; ry = 0;

L = l*(1/2)*Cl*rho*A_rudder*V*V;
D = d*(1/2)*Cd*rho*A_rudder*V*V;
Fx = -D*cos(angle_rad)+L*sin(angle_rad);
Fy = -D*sin(angle_rad)-L*cos(angle_rad);
Fz =  0;

Mx = -Fy*(rz+(a/2));
My =  Fx*(rz+(a/2));
Mz =  Fx*(b/2)*sin(angle_rad)+Fy*(rx+(a/2));

ExtForce_rudder = [Fx;Fy;Fz;Mx;My;Mz];

end

== matlab function fused_model/underwater/Control Forces1/Thruster subsystem/Thruster CP ==
  data: thrust input; thruster_torque input; ThrusterForceVector output; ang_thrust input
function ThrusterForceVector = fcn(thrust,thruster_torque,ang_thrust)

ang_rad_th = ang_thrust*(pi/180);
zth=0;%0.03;
xth=0.02;
Mth=thruster_torque;

Fx = thrust*cos(ang_rad_th);
Fy = 0;
Fz = thrust*sin(ang_rad_th);
Mx = Mth*cos(ang_rad_th);
My = Fx*zth+Fz*xth;
Mz = Mth*sin(ang_rad_th); 


ThrusterForceVector = [Fx;Fy;Fz;Mx;My;Mz];

end

== matlab function fused_model/underwater/Forces1/Coriolis Force Vector (v) ==
  data: vel input; y output
    
function y = fcn(vel)
u = vel(1);
v = vel(2);
w = vel(3);
p = vel(4);
q = vel(5);
r = vel(6);
m = 7;
Iz = 0.157;
Ix = 0.037;
Iy = 0.164;

C_rb=[0                0           0        0         m*w       -m*v;
      0                0           0       -m*w        0         m*u;
      0                0           0        m*v      -m*u         0;
      0                m*w        -m*v       0        Iz*r      -Iy*q;
      -m*w             0           m*u      -Iz*r       0        Ix*p;
      +m*v            -m*u          0         Iy*q    -Ix*p       0   ];
  
XU = -.7;
YV = -6.952;
ZW = -6.952;
KP = -0.22;
MQ = -2.22;
NR = -2.22;

C_a =  [0       0       0       0       -ZW*w   YV*v;
        0       0       0       ZW*w    0       -XU*u;
        0       0       0       -YV*v   XU*u    0;
        0       -ZW*w   YV*v    0       -NR*r   MQ*q;
        ZW*w    0       -XU*u   NR*r    0       -KP*p;
        -YV*v   XU*u    0       -MQ*q   KP*p       0];

  
% XU = -0.7;
% YV = -6.952;
% ZW = -6.952;
% KP = 0;
% MQ = -0.22;
% NR = -0.22;

% XU = -6.952;
% YV = -6.952;
% ZW = -0.7;
% KP = -0.22;
% MQ = -0.22;
% NR = 0;


% C_a =  [0       0       0       0       -XU*u   YV*v;
%         0       0       0       XU*u    0       -ZW*w;
%         0       0       0       -YV*v   ZW*w    0;
%         0       -XU*u   YV*v    0       -KP*p   MQ*q;
%         XU*u    0       -ZW*w   KP*p    0       -NR*r;
%         -YV*v   ZW*w    0       -MQ*q   NR*r       0];


   
C = C_rb+C_a;
y = C*vel;

end

== matlab function fused_model/underwater/Forces1/Damping Force Vector (v) ==
  data: vel input; y output
function y = fcn(vel)
u = vel(1);
v = vel(2);
w = vel(3);
p = vel(4);
q = vel(5);
r = vel(6);

D=  [9.46 + 3.1*abs(u) (-17.20-22.58*abs(v))/100     (28.26+607.6*abs(w))/100      0       0       0;
     0                  27.2*abs(v)      0                       0       0       -1.381;
     0                  0                       14.41+2.85*abs(w)  0       2.052 0;
     0                  0                       0                       3.05  0       0;
     0                  0                       (-3105.27+381.04*abs(w))/100  0       7.5 0;
     0                  (372.11-1006.48*abs(v))/100   0                       0       0       4.31];

y = D*vel;

end

== matlab function fused_model/underwater/Forces1/Restoring Force Vector (eta) ==
  data: eta input; y output
function y = fcn(eta)

theta = eta(5);
phi = eta(4);

W=7.7*9.81;
B=7.8*9.81;
Xg=0;
Zg=0;
Xb=0.02;
Zb=-0.03;

G=   [ (W-B)*sin(theta);
       -(W-B)*cos(theta)*sin(phi);
       -(W-B)*cos(theta)*cos(phi);
       (Zg*W-Zb*B)*cos(theta)*sin(phi);
       (Zg*W-Zb*B)*sin(theta)+(Xg*W-Xb*B)*cos(theta)*cos(phi);
       -(Xg*W-Xb*B)*cos(theta)*sin(phi)];
y =  G;

% for simulation Zb=Zg assumed
%       x           y   z
%cog	-301.22		0	89.16	(weight  ~6.8 kgs)
%cob	-308.44		0	96.30   (buoyancy 7.8 kgs)
end

== matlab function fused_model/underwater/Inverse M * Sum2 ==
  data: u input; vdot output
function vdot = fcn(u)
sum1 = u;

M_rb=[7     0      0     0       0        0;
      0     7      0     0       0        0;
      0     0      7     0       0        0;
      0     0      0     0.037   0        0;
      0     0      0     0       0.164    0;
      0     0      0     0       0        0.157];

M_a= -1*[-0.7   0       0       0       0       0;
        0      -6.952  0       0       0       0;    
        0      0       -6.952  0       0       0;
        0      0       0       0       0       0;
        0      0       0       0       -0.22   0;
        0      0       0       0       0       -0.22];

% equivalent cylinder dimension r=.06 l=.615  
M=M_rb+M_a; 
vdot = inv(M)*sum1;
end

== matlab function fused_model/underwater/Jacobian1 ==
  data: u input; eta_dot output
function eta_dot = fcn(u)

v = u(7:12); %body_frame_velocities

phi=u(4); %roll
theta=u(5); %pitch
si=u(6);   %yaw
c_p=cos(phi);
c_t=cos(theta);
c_s=cos(si);
s_p=sin(phi);
s_t=sin(theta);
s_s=sin(si);
t_t=tan(theta);


J1=[c_s*c_t    -s_s*c_p+s_p*s_t*c_s     s_s*s_p+s_t*c_s*c_p;
    s_s*c_t     c_s*c_p+s_p*s_t*s_s    -c_s*s_p+s_t*s_s*c_p;
     -s_t            s_p*c_t                 c_p*c_t       ];
       
J2=[1      s_p*t_t     c_p*t_t;
    0        c_p        -s_p;
    0      s_p/c_t     c_p/c_t ];


J=[J1 zeros(3,3); zeros(3,3) J2];
eta_dot = J * v; % y == earth_velocities

end

== matlab function fused_model/underwater/Jacobian2 ==
  data: input input; netforce_g output
function netforce_g = fcn(input)

netforce_b = input(7:12); %body_frame_velocities

phi=input(4); %roll
theta=input(5); %pitch
si=input(6);   %yaw
c_p=cos(phi);
c_t=cos(theta);
c_s=cos(si);
s_p=sin(phi);
s_t=sin(theta);
s_s=sin(si);
t_t=tan(theta);


J1=[c_s*c_t    -s_s*c_p+s_p*s_t*c_s     s_s*s_p+s_t*c_s*c_p;
    s_s*c_t     c_s*c_p+s_p*s_t*s_s    -c_s*s_p+s_t*s_s*c_p;
     -s_t            s_p*c_t                 c_p*c_t       ];
       
J2=[1      s_p*t_t     c_p*t_t;
    0        c_p        -s_p;
    0      s_p/c_t     c_p/c_t ];


J=[J1 zeros(3,3); zeros(3,3) J2];
netforce_g = J * netforce_b; % y == earth_velocities

end

== matlab function fused_model/underwater/MATLAB Function1 ==
  data: tim input; r output; lf output; rf output; th_pwm output
function [r,lf,rf,th_pwm] = fcn(tim)

if(tim >=0 && tim < 3)
    r = 0;
    lf = 0;
    rf = 0;
    th_pwm = 1500 + 200*tim/3;
elseif(tim >=3 && tim < 10)
    r = 0;
    lf = 0;
    rf = 0;
    th_pwm = 1700; 
elseif(tim >=10 && tim < 20)
    r = 0;
    lf = 30;
    rf = 30;
    th_pwm = 1700;
elseif(tim >=20 && tim < 40)
    r = 0;
    lf = -45;
    rf = -45;
    th_pwm = 1700;
elseif(tim >=40 && tim < 43)
    r = 0;
    lf = 0;
    rf = 0;
    th_pwm = 1500 + 200*(43 - tim)/3;
else
    r = 0;
    lf = 0;
    rf = 0;
    th_pwm = 1500;
end
    
end
